simulink library "Qnormalize"  (R2014b)
settings: Solver=ode45  StartTime=0.0  StopTime=10.0  RelTol=1e-3
libraries: DivisionQuatScalar x1, Qnorm x1
settings Model: Creator=Hp  LastModifiedBy=Hp

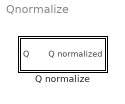
== system Qnormalize ==
  Q normalize : Subsystem

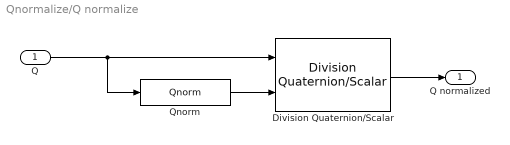
== system Qnormalize/Q normalize ==
  Q : Inport
  Division Quaternion/Scalar : DivisionQuatScalar/Division Quaternion//Scalar
  Qnorm : Qnorm/Qnorm
  Q normalized : Outport
  wires:
  Q/1 -> Qnorm/1, Division Quaternion/Scalar/1
  Division Quaternion/Scalar/1 -> Q normalized/1
  Qnorm/1 -> Division Quaternion/Scalar/2
